simulink model "model_2016a"  (Simulink 8.7)
settings: Solver=VariableStepAuto  StartTime=0.0  StopTime=25  FixedStep=0.001  RelTol=1e-5  AbsTol=1e-5
undefined symbols (not defined in the file or in its folder): control
settings Model: Creator=pmorin  LastModifiedBy=Morin  ExtModeAutoUpdateStatusClock=off
settings DataIOCC: SignalLoggingSaveFormat=ModelDataLogs
settings OptimizationCC: BooleanDataType=off  ExpressionDepthLimit=2147483647
settings DebuggingCC: SaveWithParameterizedLinksMsg=none  SignalResolutionControl=TryResolveAllWithWarning  MultiTaskDSMMsg=warning  MultiTaskCondExecSysMsg=none  FcnCallInpInsideContextMsg=EnableAllAsWarning  StateNameClashWarn=warning
settings HardwareCC: TargetUnknown=on
settings GRTTargetCC: CombineOutputUpdateFcns=off  GRTInterface=on
settings ConfigComp: CovModelRefEnable=off

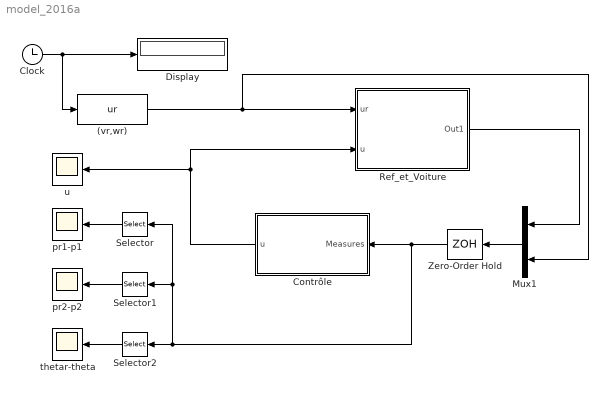
== system model_2016a ==
  (vr,wr) : MATLABFcn  MATLABFcn=ur  OutputDimensions=2
  Clock : Clock
  Contrôle : Subsystem  TreatAsAtomicUnit=on
  Display : Display
  Mux1 : Mux  Inputs=2
  Ref_et_Voiture : Subsystem  mask{init=[0;0;0;2;5;pi/4;0]}
      mask prompts: init "Initial values"
  Selector : Selector  InputPortWidth=9  IndexOptions=Index vector (dialog)  Indices=[1 4]  OutputSizes=1
  Selector1 : Selector  InputPortWidth=9  IndexOptions=Index vector (dialog)  Indices=[2 5]  OutputSizes=1
  Selector2 : Selector  InputPortWidth=9  IndexOptions=Index vector (dialog)  Indices=[3 6]  OutputSizes=1
  Zero-Order Hold : ZeroOrderHold  SampleTime=0.01
  pr1-p1 : Scope
  pr2-p2 : Scope
  thetar-theta : Scope
  u : Scope
  wires:
  Clock/1 -> (vr,wr)/1, Display/1
  Ref_et_Voiture/1(Out1) -> Mux1/1
  Contrôle/1(u) -> Ref_et_Voiture/2(u), u/1
  (vr,wr)/1 -> Mux1/2, Ref_et_Voiture/1(ur)
  Mux1/1 -> Zero-Order Hold/1
  Zero-Order Hold/1 -> Selector1/1, Selector/1, Selector2/1, Contrôle/1(Measures)
  Selector/1 -> pr1-p1/1
  Selector1/1 -> pr2-p2/1
  Selector2/1 -> thetar-theta/1

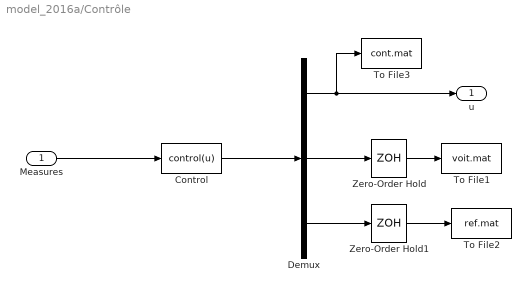
== system model_2016a/Contrôle ==
  Measures : Inport
  Control : MATLABFcn  MATLABFcn=control(u)  OutputDimensions=9
  Demux : Demux  Outputs=[2 4 3]
  To File1 : ToFile  Filename=voit.mat
  To File2 : ToFile  Filename=ref.mat
  To File3 : ToFile  Filename=cont.mat
  Zero-Order Hold : ZeroOrderHold  SampleTime=-1
  Zero-Order Hold1 : ZeroOrderHold  SampleTime=-1
  u : Outport
  wires:
  Zero-Order Hold/1 -> To File1/1
  Demux/3 -> Zero-Order Hold1/1
  Demux/2 -> Zero-Order Hold/1
  Demux/1 -> u/1, To File3/1
  Measures/1 -> Control/1
  Control/1 -> Demux/1
  Zero-Order Hold1/1 -> To File2/1

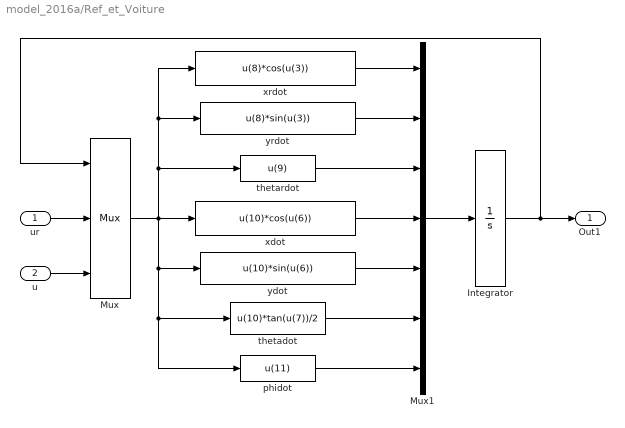
== system model_2016a/Ref_et_Voiture ==
  ur : Inport
  u : Inport  Port=2
  Integrator : Integrator  InitialCondition=init
  Mux : Mux  Inputs=[7 2 2]
  Mux1 : Mux  Inputs=7
  phidot : Fcn  Expr=u(11)
  thetadot : Fcn  Expr=u(10)*tan(u(7))/2
  thetardot : Fcn  Expr=u(9)
  xdot : Fcn  Expr=u(10)*cos(u(6))
  xrdot : Fcn  Expr=u(8)*cos(u(3))
  ydot : Fcn  Expr=u(10)*sin(u(6))
  yrdot : Fcn  Expr=u(8)*sin(u(3))
  Out1 : Outport
  wires:
  ur/1 -> Mux/2
  Integrator/1 -> Out1/1, Mux/1
  Mux1/1 -> Integrator/1
  Mux/1 -> thetardot/1, yrdot/1, xrdot/1, ydot/1, thetadot/1, phidot/1, xdot/1
  u/1 -> Mux/3
  phidot/1 -> Mux1/7
  thetadot/1 -> Mux1/6
  ydot/1 -> Mux1/5
  xdot/1 -> Mux1/4
  thetardot/1 -> Mux1/3
  xrdot/1 -> Mux1/1
  yrdot/1 -> Mux1/2
